simulink model "CAG_3PH"  (R2020a)
settings: Solver=FixedStepAuto  StartTime=0.0  StopTime=10  FixedStep=1e-6  RelTol=1e-3  EnableMultiTasking=on
libraries: powerlib x14
settings Model: SimulationMode=accelerator  Creator=SINA  LastModifiedBy=ABO-CHIFA
settings DataIOCC: ReturnWorkspaceOutputs=off
settings OptimizationCC: LifeSpan=inf
settings DebuggingCC: SFUnexpectedBacktrackingDiag=warning  SFNoUnconditionalDefaultTransitionDiag=warning  ArithmeticOperatorsInVariantConditions=warning
settings SFSimCC: SimUseLocalCustomCode=off  CustomCodeUndefinedFunction=UseInterfaceOnly
settings RTWCC: RTWUseLocalCustomCode=off
settings CodeAppCC: StateflowObjectComments=on
settings GRTTargetCC: TargetLangStandard=C89/C90 (ANSI)
settings ConfigComp: CovMetricSettings=dw  CovHtmlReporting=on  CovSaveCumulativeToWorkspaceVar=on  CovSaveSingleToWorkspaceVar=on  CovExternalEMLEnable=off
settings SimscapeCC: SimscapeNormalizeSystem=off

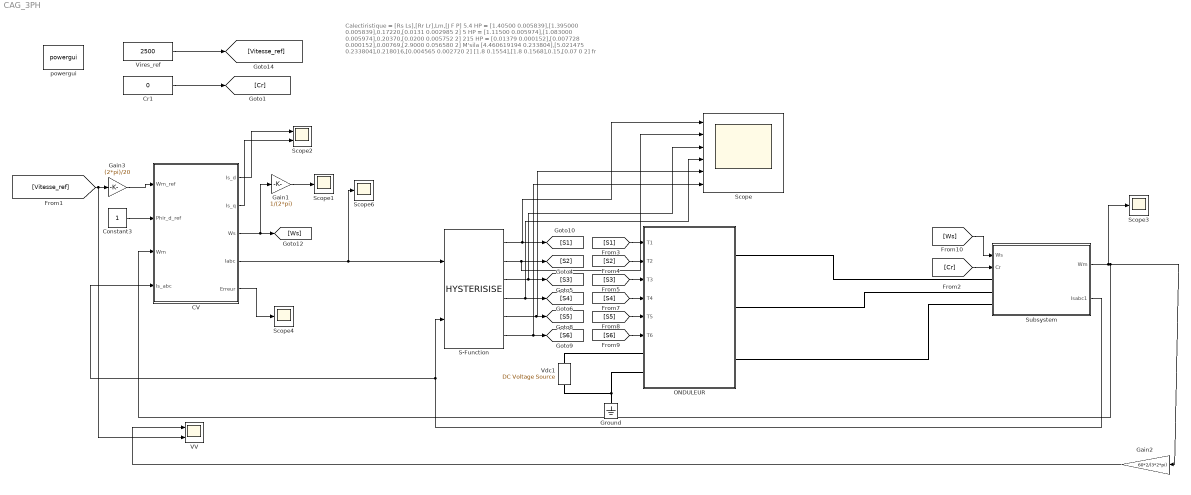
== system CAG_3PH ==
  note: Calectiristique = [Rs Ls],[Rr Lr],Lm,[J F P]
      |
      | 5.4 HP = [1.40500 0.005839],[1.395000 0.005839],0.17220,[0.0131 0.002985 2]
      | 5 HP = [1.11500 0.005974],[1.083000 0.005974],0.20370,[0.0200 0.005752 2]
      | 215 HP = [0.01379 0.000152],[0.007728 0.000152],0.00769,[2.9000 0.056580 2]
      |
      | M'sila
      | [4.460619194 0.233804],[5.021475 0.233804],0.218016,[0.004565 0.002720 2]
      |
      | [1.8 0.1554],[1.8 0.1568],0.15,[0.07 0 2] fr
  CV : Subsystem
  Constant3 : Constant
  Cr1 : Constant  Value=0
  Gain1 : Gain  Gain=1/(2*pi)
  Gain2 : Gain  Gain=60*2/(3*2*pi)
  Gain3 : Gain  Gain=(2*pi)/20
  Ground : powerlib/Elements/Ground  LConnTagsString=a
  ONDULEUR : Subsystem
  S-Function : S-Function  FunctionName=HYSTERISISE  SFunctionDeploymentMode=off  EnableBusSupport=off
  Scope : Scope  NumInputPorts=6
  Scope{1,3..4,6} (4 alike) : Scope
  Scope2 : Scope  NumInputPorts=2
  Subsystem : Subsystem
  VV : Scope  NumInputPorts=2
  Vdc1 : powerlib/Electrical Sources/DC Voltage Source  Amplitude=650  Measurements=Voltage
  Vires_ref : Constant  Value=2500
  powergui : powerlib/powergui  Priority=1  SimulationMode=Discrete  SampleTime=1e-6  frequency=60  Iterations=50  frequencyindice=0  Pbase=100e6  ErrMax=1e-4  UnitsV=kV  UnitsW=MW  buscounter=0  FunctionMessages=off  echomessages=off  EnableUseOfTLC=off  CurrentSourceSwitches=off  DisableSnubberDevices=off  DisableRonSwitches=off  DisableVfSwitches=off  DisplayEquations=off  AutomaticDiscreteSolvers=off  SolverType=Tustin/Backward Euler (TBE)  Interpol=off  ExternalGateDelay=off  methode=off  Ts=0  x0status=blocks  SPID=off  SwTol=0  HookPort=off  NonlinearTolerance=1e-4  nMaxIteration=100  ContinueOnMaxIteration=off  RestoreLinks=warning  ResistiveCurrentMeasurement=off  Frange=[0:2:500]  Ylog=off  Xlog=on  ShowGrid=off  save=off  variable=ZData  structure=0  ZoomFFT=on  StartTime=0.0  cycles=1  DisplayStyle=1  fundamental=60  FreqAxis=off  MaxFrequency=1000  frequencyindicesteady=1  RmsSteady=1  display=off
  wires:
  Constant3/1 -> CV/2(Phir_d_ref)
  CV/3(Ws) -> [Ws], Gain1/1
  CV/4(Iabc) -> Scope6/1, S-Function/1
  Gain1/1 -> Scope1/1
  CV/1(Is_d) -> Scope2/1
  CV/2(Is_q) -> Scope2/2
  CV/5(Erreur) -> Scope4/1
  Cr1/1 -> [Cr]
  [Ws] -> Subsystem/1(Ws)
  [Cr] -> Subsystem/2(Cr)
  [S1] -> ONDULEUR/1("T1 ")
  [S3] -> ONDULEUR/3("T3  ")
  [S5] -> ONDULEUR/5("T5 ")
  [S2] -> ONDULEUR/2("T2 ")
  [S4] -> ONDULEUR/4("T4 ")
  [S6] -> ONDULEUR/6("T6 ")
  S-Function/5 -> Scope/5, [S5]
  S-Function/4 -> Scope/4, [S4]
  S-Function/3 -> Scope/3, [S3]
  S-Function/2 -> Scope/2, [S2]
  S-Function/1 -> Scope/1, [S1]
  S-Function/6 -> Scope/6, [S6]
  [Vitesse_ref] -> VV/2, Gain3/1
  Gain3/1 -> CV/1(Wm_ref)
  Gain2/1 -> VV/1
  Subsystem/2(Isabc1) -> CV/4(Is_abc), S-Function/2
  Subsystem/1(Wm) -> Scope3/1, CV/3(Wm), Gain2/1
  Vires_ref/1 -> [Vitesse_ref]
  connections:
  Vdc1/RConn1 -- ONDULEUR/LConn1
  Ground/LConn1 -- ONDULEUR/LConn2 -- Vdc1/LConn1
  Subsystem/LConn1 -- ONDULEUR/RConn1
  Subsystem/LConn2 -- ONDULEUR/RConn2
  Subsystem/LConn3 -- ONDULEUR/RConn3

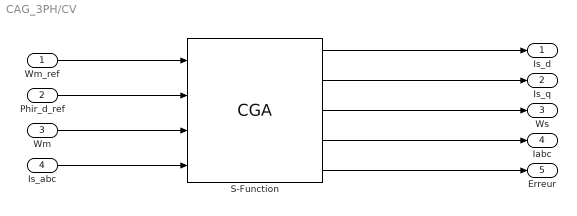
== system CAG_3PH/CV ==
  Wm_ref : Inport
  Phir_d_ref : Inport  Port=2
  Wm : Inport  Port=3
  Is_abc : Inport  Port=4
  S-Function : S-Function  FunctionName=CGA  Parameters=[1.40500 0.005839],[1.395000 0.005839],0.17220,[0.0131 0.002985 2]  SFunctionDeploymentMode=off  EnableBusSupport=off
  Is_d : Outport
  Is_q : Outport  Port=2
  Ws : Outport  Port=3
  Iabc : Outport  Port=4
  Erreur : Outport  Port=5
  wires:
  S-Function/4 -> Iabc/1
  S-Function/3 -> Ws/1
  S-Function/2 -> Is_q/1
  S-Function/1 -> Is_d/1
  Wm/1 -> S-Function/3
  Phir_d_ref/1 -> S-Function/2
  Wm_ref/1 -> S-Function/1
  S-Function/5 -> Erreur/1
  Is_abc/1 -> S-Function/4

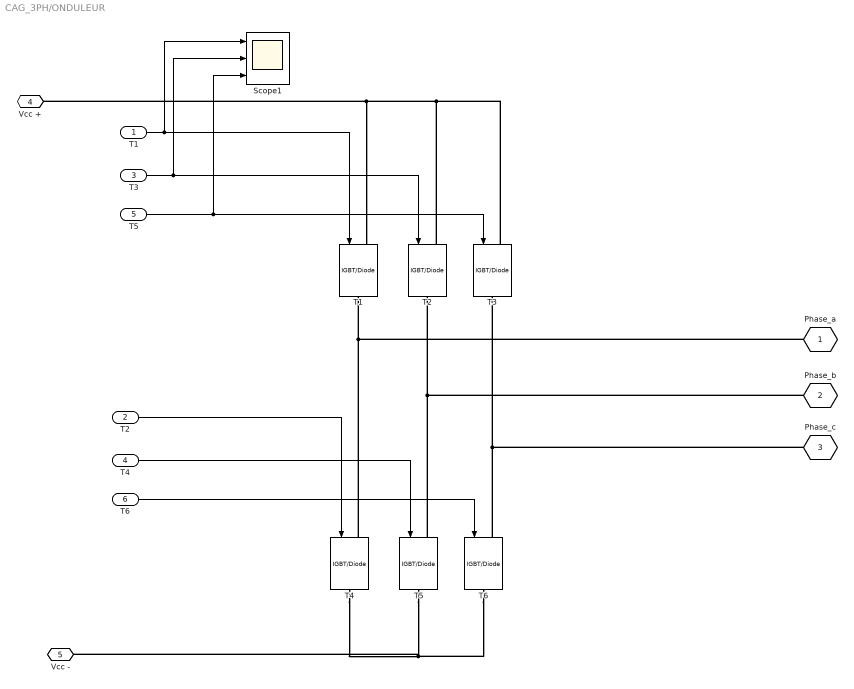
== system CAG_3PH/ONDULEUR ==
  "T1 " : Inport
  "T2 " : Inport  Port=2
  "T3  " : Inport  Port=3
  "T4 " : Inport  Port=4
  "T5 " : Inport  Port=5
  "T6 " : Inport  Port=6
  Scope1 : Scope  NumInputPorts=3
  T{1..6} (6 alike) : powerlib/Power Electronics/IGBT//Diode  Ron=1e-3  Rs=1e5  Cs=inf  Measurements=off
  Phase_a : PMIOPort  Tag=PMCPort  Side=Right
  Phase_b : PMIOPort  Tag=PMCPort  Port=2  Side=Right
  Phase_c : PMIOPort  Tag=PMCPort  Port=3  Side=Right
  Vcc + : PMIOPort  Port=4  Side=Left
  Vcc - : PMIOPort  Port=5  Side=Left
  wires:
  "T1 "/1 -> Scope1/1, T1/1
  "T3  "/1 -> Scope1/2, T2/1
  "T5 "/1 -> Scope1/3, T3/1
  "T2 "/1 -> T4/1
  "T4 "/1 -> T5/1
  "T6 "/1 -> T6/1
  connections:
  T2/LConn1 -- T3/LConn1 -- Vcc +/RConn1 -- T1/LConn1
  T5/RConn1 -- T4/RConn1 -- Vcc -/RConn1 -- T6/RConn1
  T4/LConn1 -- Phase_a/RConn1 -- T1/RConn1
  T5/LConn1 -- Phase_b/RConn1 -- T2/RConn1
  T6/LConn1 -- Phase_c/RConn1 -- T3/RConn1

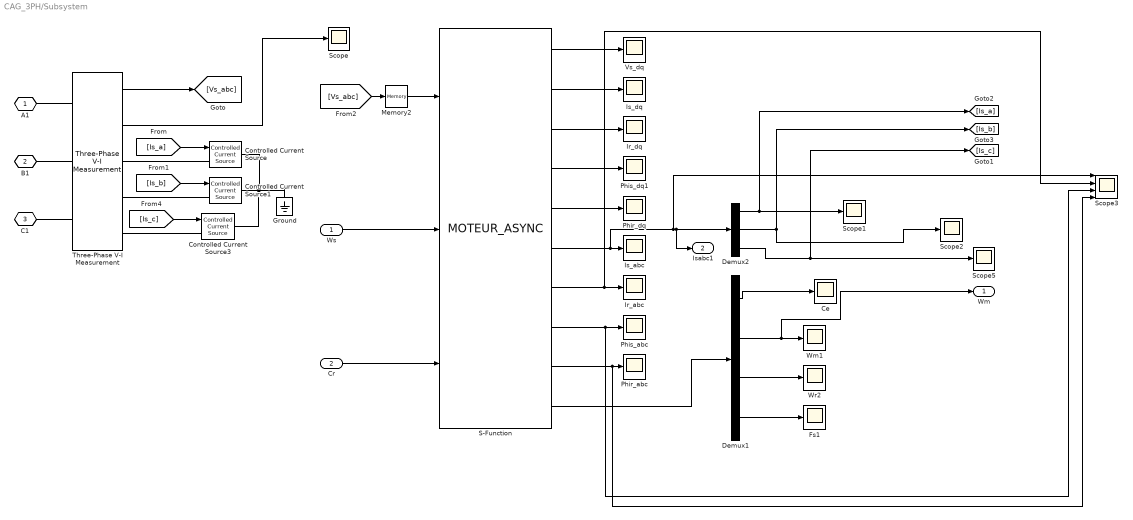
== system CAG_3PH/Subsystem ==
  Ws : Inport
  Cr : Inport  Port=2
  Ce : Scope
  Controlled Current Source : powerlib/Electrical Sources/Controlled Current Source  Initialize=off  Source_Type=AC  Amplitude=0  Phase=0  Frequency=50  Measurements=Current
  Controlled Current Source1 : powerlib/Electrical Sources/Controlled Current Source  Initialize=off  Source_Type=AC  Amplitude=0  Phase=0  Frequency=50  Measurements=Current
  Controlled Current Source3 : powerlib/Electrical Sources/Controlled Current Source  Initialize=off  Source_Type=AC  Amplitude=0  Phase=0  Frequency=50  Measurements=Current
  Demux1 : Demux
  Demux2 : Demux  Outputs=3
  Fs1 : Scope
  Ground : powerlib/Elements/Ground  LConnTagsString=a
  Ir_abc : Scope
  Ir_dq : Scope
  Is_abc : Scope
  Is_dq : Scope
  Memory2 : Memory
  Phir_abc : Scope
  Phir_dq : Scope
  Phis_abc : Scope
  Phis_dq1 : Scope
  S-Function : S-Function  FunctionName=MOTEUR_ASYNC  Parameters=[1.40500 0.005839],[1.395000 0.005839],0.17220,[0.0131 0.002985 2]  SFunctionDeploymentMode=off  EnableBusSupport=off
  Scope{,1..2,5} (4 alike) : Scope
  Scope3 : Scope  NumInputPorts=4
  Three-Phase V-I Measurement : powerlib/Measurements/Three-Phase V-I Measurement  VoltageMeasurement=phase-to-ground  SetLabelV=off  LabelV=Vabc  Vpu=off  VpuLL=off  CurrentMeasurement=yes  SetLabelI=off  LabelI=Iabc  Ipu=off  Pbase=100e6  Vbase=500e3  OutputType=Complex  PhasorSimulation=off  PSBequivalent=0
  Vs_dq : Scope
  Wm1 : Scope
  Wr2 : Scope
  A1 : PMIOPort  Tag=PMCPort  Side=Left
  B1 : PMIOPort  Tag=PMCPort  Port=2  Side=Left
  C1 : PMIOPort  Tag=PMCPort  Port=3  Side=Left
  Wm : Outport
  Isabc1 : Outport  Port=2
  wires:
  Demux2/3 -> [Is_c], Scope5/1
  Demux1/2 -> Wm/1, Wm1/1
  Demux1/3 -> Wr2/1
  Ws/1 -> S-Function/2
  S-Function/7 -> Scope3/2, Ir_abc/1
  S-Function/9 -> Scope3/4, Phir_abc/1
  S-Function/2 -> Is_dq/1
  Demux1/4 -> Fs1/1
  S-Function/6 -> Scope3/1, Isabc1/1, Demux2/1, Is_abc/1
  Demux1/1 -> Ce/1
  S-Function/5 -> Phir_dq/1
  S-Function/10 -> Demux1/1
  S-Function/8 -> Scope3/3, Phis_abc/1
  S-Function/4 -> Phis_dq1/1
  S-Function/1 -> Vs_dq/1
  Cr/1 -> S-Function/3
  S-Function/3 -> Ir_dq/1
  [Is_a] -> Controlled Current Source/1
  [Is_b] -> Controlled Current Source1/1
  Three-Phase V-I Measurement/1 -> [Vs_abc]
  Demux2/2 -> Scope2/1, [Is_b]
  Demux2/1 -> Scope1/1, [Is_a]
  [Vs_abc] -> Memory2/1
  Memory2/1 -> S-Function/1
  Three-Phase V-I Measurement/2 -> Scope/1
  [Is_c] -> Controlled Current Source3/1
  connections:
  Controlled Current Source/RConn1 -- Controlled Current Source3/RConn1 -- Controlled Current Source1/RConn1 -- Ground/LConn1
  Three-Phase V-I Measurement/RConn2 -- Controlled Current Source1/LConn1
  Three-Phase V-I Measurement/RConn1 -- Controlled Current Source/LConn1
  A1/RConn1 -- Three-Phase V-I Measurement/LConn1
  B1/RConn1 -- Three-Phase V-I Measurement/LConn2
  C1/RConn1 -- Three-Phase V-I Measurement/LConn3
  Three-Phase V-I Measurement/RConn3 -- Controlled Current Source3/LConn1
